simulink model "canudas_goal"  (R2012b)
settings: Solver=FixedStepDiscrete  StartTime=0.0  StopTime=Inf  FixedStep=0.033  RelTol=1e-3
values from neighbouring files (symbols this model uses):
  eps1 = 0.05    [param.m]
  eps2 = 2*pi*5/360    (= 0.0872664625997)    [param.m]
  K1 = 1.35    [param.m]
  K2 = 4.6    [param.m]
  thetar = pi    (= 3.14159265359)    [param.m]
  xr = 0    [param.m]
  yr = 0    [param.m]
libraries: simiam x5, simulink x3
settings Model: Creator=jdelacroix  LastModifiedBy=samati
settings DataIOCC: SignalLoggingSaveFormat=ModelDataLogs  SaveOutput=off  SaveTime=off
settings DebuggingCC: MultiTaskDSMMsg=warning  MultiTaskCondExecSysMsg=none  FcnCallInpInsideContextMsg=EnableAllAsWarning  StrictBusMsg=None
settings RTWCC: IncludeERTFirstTime=on
settings CodeAppCC: CustomSymbolStrType=$N$R$M_T  InternalIdentifier=Shortened
settings GRTTargetCC: CodeReplacementLibrary=None  CPPClassGenCompliant=on

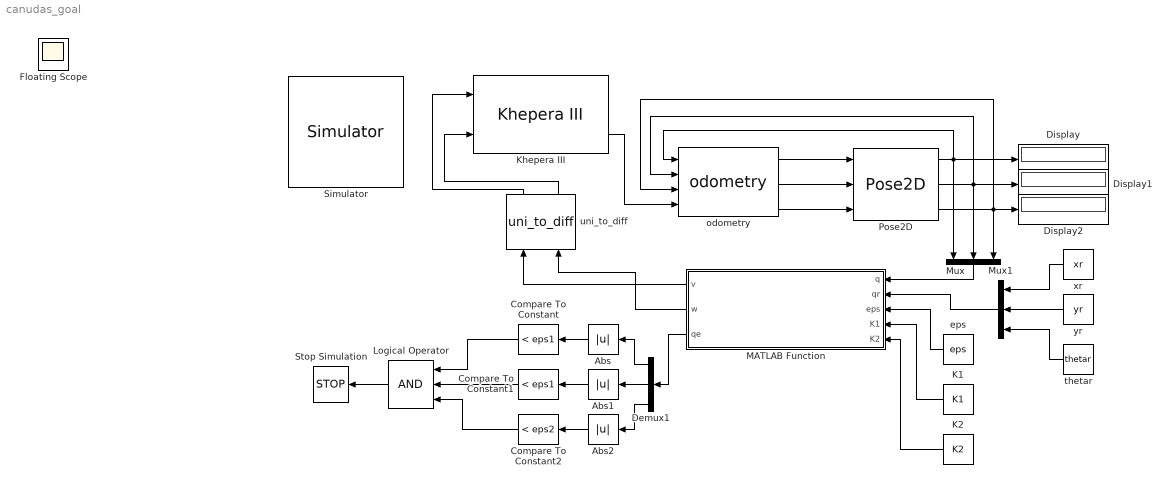
== system canudas_goal ==
  Abs : Abs
  Abs1 : Abs
  Abs2 : Abs
  Compare To Constant : simulink/Logic and Bit Operations/Compare To Constant  relop=<  const=eps1  OutDataTypeStr=boolean
  Compare To Constant1 : simulink/Logic and Bit Operations/Compare To Constant  relop=<  const=eps1  OutDataTypeStr=boolean
  Compare To Constant2 : simulink/Logic and Bit Operations/Compare To Constant  relop=<  const=eps2  OutDataTypeStr=boolean
  Demux1 : Demux  Outputs=3
  Display : Display
  Display1 : Display
  Display2 : Display
  K1 : Constant  Value=K1
  K2 : Constant  Value=K2
  Khepera III : simiam/Khepera III  x_0=0  y_0=0  theta_0=0  robot_id=1
  Logical Operator : Logic  Inputs=3  AllPortsSameDT=off  OutDataTypeStr=boolean
  MATLAB Function : MATLAB Function  TreatAsAtomicUnit=on
  Mux : Mux  Inputs=3
  Mux1 : Mux  Inputs=3
  Pose2D : simiam/Pose2D  SystemSampleTime=-1
  Simulator : simiam/Simulator  Priority=1
  Stop Simulation : Stop
  eps : Constant  Value=eps
  odometry : simiam/odometry  wheel_radius=r  wheel_base_length=l  ticks_per_rev=2675
  thetar : Constant  Value=thetar
  uni_to_diff : simiam/uni_to_diff  wheel_radius=r  wheel_base_length=l
  xr : Constant  Value=xr
  yr : Constant  Value=yr
  Floating Scope : Scope
  wires:
  uni_to_diff/1 -> Khepera III/1
  uni_to_diff/2 -> Khepera III/2
  odometry/2 -> Pose2D/2
  odometry/1 -> Pose2D/1
  Khepera III/2 -> odometry/4
  Pose2D/1 -> Display/1, Mux/1, odometry/1
  Pose2D/2 -> Display1/1, odometry/2, Mux/2
  Pose2D/3 -> Display2/1, odometry/3, Mux/3
  odometry/3 -> Pose2D/3
  xr/1 -> Mux1/1
  yr/1 -> Mux1/2
  thetar/1 -> Mux1/3
  Mux/1 -> MATLAB Function/1(q)
  Mux1/1 -> MATLAB Function/2(qr)
  MATLAB Function/2(w) -> uni_to_diff/2
  MATLAB Function/3(qe) -> Demux1/1
  Logical Operator/1 -> Stop Simulation/1
  Compare To Constant1/1 -> Logical Operator/2
  Compare To Constant/1 -> Logical Operator/1
  Compare To Constant2/1 -> Logical Operator/3
  eps/1 -> MATLAB Function/3(eps)
  MATLAB Function/1(v) -> uni_to_diff/1
  K1/1 -> MATLAB Function/4(K1)
  K2/1 -> MATLAB Function/5(K2)
  Demux1/1 -> Abs/1
  Abs/1 -> Compare To Constant/1
  Demux1/2 -> Abs1/1
  Abs1/1 -> Compare To Constant1/1
  Abs2/1 -> Compare To Constant2/1
  Demux1/3 -> Abs2/1

== matlab function canudas_goal/MATLAB Function ==
  data: q input; v output; w output; qr input; qe output; eps input; K1 input; K2 input
function [v, w, qe] = canudas_goal(q, qr, eps, K1, K2)
           
% Error
T = [cos(qr(3)), sin(qr(3)), 0;...
     -sin(qr(3)), cos(qr(3)), 0;...
     0, 0, 1];
qe = T*(q-qr);

% Compute initial z state
% there are some tests to ensure continuity (inf points)
% atan2 certifiates that the angle stazs in [-pi, pi]
if((abs(qe(1))<eps) && (abs(qe(2))==eps))
    thetad = 0;
else
    thetad = 2*atan2(qe(2),qe(1));
    thetad = limit_angle(thetad);
end

if(abs(qe(2))<eps)
    r = 0;
else
    r = (qe(1)^2 + qe(2)^2)/(2*qe(2));
end

a = r * thetad;
alpha = qe(3)-thetad;
alpha = limit_angle(alpha);

% Compute commands
G = [cos(q(3)), 0;...
     sin(q(3)), 0;...
     0, 1];

J = [thetad*qe(1)/qe(2) - 1, thetad*(1-qe(1)^2/qe(2)^2)/2 + qe(1)/qe(2), 0;...
     2*qe(2)/(1+qe(2)^2/qe(1)^2)/qe(1)^2, -2/(1+qe(2)^2/qe(1)^2)/qe(1), 1];
      
B = J*T*G;

v = -K1*B(1,1)*a;
w = -B(2,1)*v - K2*alpha;

end
